simulink model "diffDrive"  (R2023a)
settings: Solver=VariableStepAuto  StartTime=0.0  StopTime=1  RelTol=1e-3
values from neighbouring files (symbols this model uses):
  ax = 0.1    [playground2.m]    (also in process_sim.m = [0, 0, 0.5, 0.5, 0.5, 0, 0, 0, -0.5, -0.5, -0.5])
  ax0 = 0    [process_sim.m]
  ay = 0.5    [playground2.m]    (also in process_sim.m = [0.25, 0.25, 0.25, 0.25, 0, 0, 0, 0, -0.75, -0.75, -0.75])
  ay0 = 0    [process_sim.m]
  fullX0 = [x0; y0; atan2(vy0, vx0); sqrt(vx0^2 + vy0^2); 0]    [playground2.m]    (also in process_sim.m = [x0; y0; atan2(vy0, vx0); sqrt(vx0^2 + vy0^2); 0] + delta)
  input_order = 2    [process_sim.m]
  jx = [0, 0, 1, 1, 1, -1, -1, -1, 0, 0, 0, -1, -1, -1, 1, 1, 1]    [process_sim.m]
  jy = [1, 1, 1, -1, -1, 0, 0, 0, -1, -1, -1, 1, 1, 1, 0, 0, 0]    [process_sim.m]
  T = 3    [playground.m]    (also in playground2.m = 0.1; predictiveControl.m = 0.1; process_sim.m = 0.1)
  vx0 = 0.5    [playground2.m]    (also in process_sim.m)
  vy0 = 0    [playground2.m]    (also in process_sim.m)
  x0 = x_lin + [0.01; -0.01; 0.02; 0.01; 0.001]    [playground.m]    (also in playground2.m = 0; process_sim.m = 0)
  y0 = 0    [playground2.m]    (also in process_sim.m)
settings Model: Creator=wcompton  LastModifiedBy=wcompton

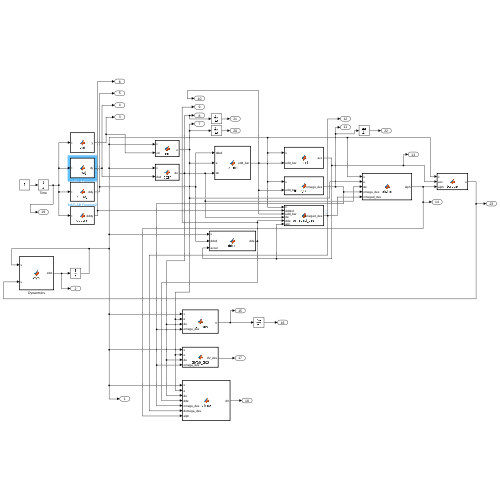
[thumbnail: Simulink's stored preview of the top-level diagram]
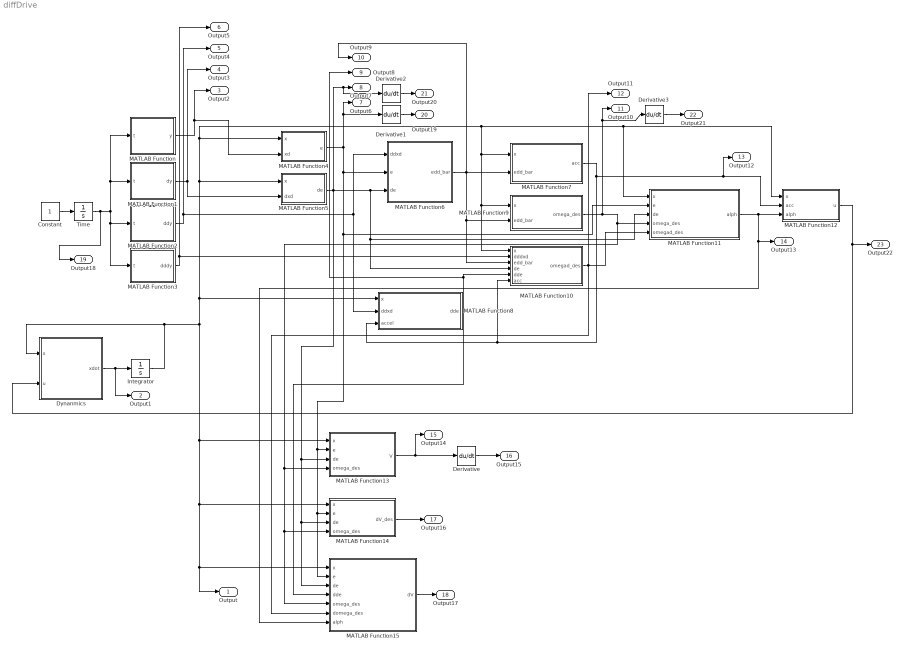
== system diffDrive ==
  Constant : Constant
  Derivative{,1..3} (4 alike) : Derivative
  Dynanmics : MATLAB Function  TreatAsAtomicUnit=on
  Integrator : Integrator  InitialCondition=fullX0
  MATLAB Function : MATLAB Function  TreatAsAtomicUnit=on
  MATLAB Function1 : MATLAB Function  TreatAsAtomicUnit=on
  MATLAB Function10 : MATLAB Function  TreatAsAtomicUnit=on
  MATLAB Function11 : MATLAB Function  TreatAsAtomicUnit=on
  MATLAB Function12 : MATLAB Function  TreatAsAtomicUnit=on
  MATLAB Function13 : MATLAB Function  TreatAsAtomicUnit=on
  MATLAB Function14 : MATLAB Function  TreatAsAtomicUnit=on
  MATLAB Function15 : MATLAB Function  TreatAsAtomicUnit=on
  MATLAB Function2 : MATLAB Function  TreatAsAtomicUnit=on
  MATLAB Function3 : MATLAB Function  TreatAsAtomicUnit=on
  MATLAB Function4 : MATLAB Function  TreatAsAtomicUnit=on
  MATLAB Function5 : MATLAB Function  TreatAsAtomicUnit=on
  MATLAB Function6 : MATLAB Function  TreatAsAtomicUnit=on
  MATLAB Function7 : MATLAB Function  TreatAsAtomicUnit=on
  MATLAB Function8 : MATLAB Function  TreatAsAtomicUnit=on
  MATLAB Function9 : MATLAB Function  TreatAsAtomicUnit=on
  Time : Integrator
  Output : Outport
  Output1 : Outport  Port=2
  Output2 : Outport  Port=3
  Output3 : Outport  Port=4
  Output4 : Outport  Port=5
  Output5 : Outport  Port=6
  Output6 : Outport  Port=7
  Output7 : Outport  Port=8
  Output8 : Outport  Port=9
  Output9 : Outport  Port=10
  Output10 : Outport  Port=11
  Output11 : Outport  Port=12
  Output12 : Outport  Port=13
  Output13 : Outport  Port=14
  Output14 : Outport  Port=15
  Output15 : Outport  Port=16
  Output16 : Outport  Port=17
  Output17 : Outport  Port=18
  Output18 : Outport  Port=19
  Output19 : Outport  Port=20
  Output20 : Outport  Port=21
  Output21 : Outport  Port=22
  Output22 : Outport  Port=23
  wires:
  Dynanmics/1(xdot) -> Integrator/1, Output1/1
  Integrator/1 -> MATLAB Function14/1(x), Output/1, MATLAB Function15/1(x), MATLAB Function13/1(x), MATLAB Function4/1(x), MATLAB Function9/1(x), MATLAB Function10/1(x), MATLAB Function7/1(x), MATLAB Function11/1(x), MATLAB Function12/1(x), MATLAB Function5/1(x), MATLAB Function8/1(x), Dynanmics/1(x)
  Constant/1 -> Time/1
  Time/1 -> Output18/1, MATLAB Function3/1(t), MATLAB Function2/1(t), MATLAB Function/1(t), MATLAB Function1/1(t)
  MATLAB Function/1(y) -> MATLAB Function4/2(xd), Output2/1
  MATLAB Function1/1(dy) -> Output3/1, MATLAB Function5/2(dxd)
  MATLAB Function4/1(e) -> MATLAB Function13/2(e), MATLAB Function15/2(e), MATLAB Function14/2(e), MATLAB Function11/2(e), MATLAB Function6/2(e), Derivative1/1, Output6/1
  MATLAB Function5/1(de) -> MATLAB Function6/3(de), MATLAB Function10/4(de), MATLAB Function11/3(de), Derivative2/1, Output7/1, MATLAB Function14/3(de), MATLAB Function15/3(de), MATLAB Function13/3(de)
  MATLAB Function2/1(ddy) -> Output4/1, MATLAB Function6/1(ddxd), MATLAB Function8/2(ddxd)
  MATLAB Function6/1(edd_bar) -> Output9/1, MATLAB Function9/2(edd_bar), MATLAB Function10/3(edd_bar), MATLAB Function7/2(edd_bar)
  MATLAB Function7/1(acc) -> MATLAB Function8/3(accel), MATLAB Function10/6(acc), Output12/1, MATLAB Function12/2(acc)
  MATLAB Function8/1(dde) -> MATLAB Function15/4(dde), MATLAB Function10/5(dde), Output8/1
  MATLAB Function9/1(omega_des) -> MATLAB Function11/4(omega_des), MATLAB Function13/4(omega_des), MATLAB Function14/4(omega_des), MATLAB Function15/5(omega_des), Output10/1, Derivative3/1
  MATLAB Function10/1(omegad_des) -> MATLAB Function15/6(domega_des), MATLAB Function11/5(omegad_des), Output11/1
  MATLAB Function11/1(alph) -> MATLAB Function15/7(alph), Output13/1, MATLAB Function12/3(alph)
  MATLAB Function12/1(u) -> Output22/1, Dynanmics/2(u)
  MATLAB Function13/1(V) -> Output14/1, Derivative/1
  MATLAB Function3/1(dddy) -> MATLAB Function10/2(dddxd), Output5/1
  MATLAB Function15/1(dV) -> Output17/1
  MATLAB Function14/1(dV_des) -> Output16/1
  Derivative/1 -> Output15/1
  Derivative1/1 -> Output19/1
  Derivative2/1 -> Output20/1
  Derivative3/1 -> Output21/1

== matlab function diffDrive/MATLAB Function6 ==
  data: ddxd input; edd_bar output; e input; de input; params parameter
function edd_bar = des_dde(ddxd, e, de, params)

edd_bar = ddxd - params.Kp * e - params.Kd * de;

== matlab function diffDrive/MATLAB Function7 ==
  data: x input; acc output; edd_bar input
function acc = accel(x, edd_bar)

acc = [cos(x(3)), sin(x(3))] * edd_bar;

== matlab function diffDrive/MATLAB Function8 ==
  data: x input; dde output; ddxd input; accel input
function dde = dderr(x, ddxd, accel)

dde = - ddxd + [cos(x(3)), -x(4) * sin(x(3)); sin(x(3)), x(4) * cos(x(3))] * [accel; x(5)];

== matlab function diffDrive/MATLAB Function9 ==
  data: x input; omega_des output; edd_bar input
function omega_des = omega_des(x, edd_bar)

omega_des = [-1 / x(4) * sin(x(3)), 1 / x(4) * cos(x(3))] * edd_bar;

== matlab function diffDrive/MATLAB Function10 ==
  data: x input; dddxd input; omegad_des output; edd_bar input; de input; dde input; acc input; params parameter
function omegad_des = omegad_des(x, dddxd, edd_bar, de, dde, acc, params)

omegad_des = [acc / x(4)^2 * sin(x(3)) - x(5) / x(4) * cos(x(3)), -acc / x(4)^2 * cos(x(3)) - x(5) / x(4) * sin(x(3))] * edd_bar + [-1 / x(4) * sin(x(3)), 1 / x(4) * cos(x(3))] * (dddxd - params.Kp * de - params.Kd * dde);

== matlab function diffDrive/MATLAB Function11 ==
  data: x input; e input; de input; alph output; omega_des input; omegad_des input; params parameter
function alph = alpha(x, e, de, omega_des, omegad_des, params)

alph = -params.sigma / 2 * (x(5) - omega_des) + omegad_des - 2 * [e', de'] * params.P * [0; 0; -x(4) * sin(x(3)); x(4) * cos(x(3))];

== matlab function diffDrive/MATLAB Function12 ==
  data: x input; u output; acc input; alph input; params parameter
function u = torque(x, acc, alph, params)

u = accelToTorque(x, [acc; alph], params);

== matlab function diffDrive/MATLAB Function13 ==
  data: x input; V output; e input; de input; omega_des input; params parameter
function V = laypunov(x, e, de, omega_des, params)

Ve = [e; de]' * params.P * [e; de];
V = Ve + 0.5 * (omega_des - x(5)).^2;

== matlab function diffDrive/MATLAB Function14 ==
  data: x input; dV_des output; e input; de input; omega_des input; params parameter
function dV_des = dlyap_des(x, e, de, omega_des, params)

dVe = -[e; de]' * [e; de];
dV_des = dVe - params.sigma / 2 * (omega_des - x(5)).^2;

== matlab function diffDrive/MATLAB Function ==
  data: t input; y output; x0 parameter; vx0 parameter; ax0 parameter; y0 parameter; vy0 parameter; ay0 parameter; T parameter; ax parameter; ay parameter; jx parameter; jy parameter; input_order parameter
function y = traj(t, x0, vx0, ax0, y0, vy0, ay0, T, ax, ay, jx, jy, input_order)
if input_order == 2
    ind = 1;
    while t > T
        x0 = x0 + vx0 * T + 0.5 * ax(ind) * T^2;
        vx0 = vx0 + ax(ind) * T;
        y0 = y0 + vy0 * T + 0.5 * ay(ind) * T^2;
        vy0 = vy0 + ay(ind) * T;
        t = t - T;
        ind = ind + 1;
    end
    y = [x0 + vx0 * t + 0.5 * ax(ind) * t^2;y0 + vy0 * t + 0.5 * ay(ind) * t^2];
elseif input_order == 3
    ind = 1;
    while t > T
        x0 = x0 + vx0 * T + 0.5 * ax0 * T^2 + 1/6 * jx(ind) * T^3;
        vx0 = vx0 + ax0 * T + 0.5 * jx(ind) * T^2;
        ax0 = ax0 + jx(ind) * T;
        y0 = y0 + vy0 * T + 0.5 * ay0 * T^2 + 1/6 * jy(ind) * T^3;
        vy0 = vy0 + ay0 * T + 0.5 * jy(ind) * T^2;
        ay0 = ay0 + jy(ind) * T;
        t = t - T;
        ind = ind + 1;
    end
    y = [x0 + vx0 * t + 0.5 * ax0 * t^2 + jx(ind) / 6 * t^3; y0 + vy0 * t + 0.5 * ay0 * t^2 + jy(ind) / 6 * t^3];
else
    y = [0; 0];
end

== matlab function diffDrive/MATLAB Function15 ==
  data: x input; dV output; e input; de input; dde input; omega_des input; domega_des input; alph input; params parameter
function dV = dlyap(x, e, de, dde, omega_des, domega_des, alph, params)

dV = 2 * [de; dde]' * params.P * [e; de] + (omega_des - x(5)) * (domega_des - alph);

== matlab function diffDrive/Dynanmics ==
  data: x input; u input; xdot output; params parameter
function xdot = dyn(x, u, params)

th = x(3);
v = x(4);
w = x(5);
R = params.R;
L = params.L;
alpha = params.m + 2 * params.Iw / R.^2;
beta = params.I + 2 * L^.2 / R.^2 * params.Iw;
mcd = params.mc * params.d;

tr = u(1);
tl = u(2);

xdot = [
    v * cos(th);
    v * sin(th);
    w;
    (mcd * w.^2 + (tr + tl) / R) / alpha;
    (-mcd * w * v + (tr - tl) * L / R) / beta
];

== matlab function diffDrive/MATLAB Function1 ==
  data: t input; dy output; vx0 parameter; ax0 parameter; vy0 parameter; ay0 parameter; T parameter; ax parameter; ay parameter; jx parameter; jy parameter; input_order parameter
function dy = dtraj(t, vx0, ax0, vy0, ay0, T, ax, ay, jx, jy, input_order)
if input_order == 2
    ind = 1;
    while t > T
        vx0 = vx0 + ax(ind) * T;
        vy0 = vy0 + ay(ind) * T;
        t = t - T;
        ind = ind + 1;
    end
    dy = [vx0 + ax(ind) * t; vy0 + ay(ind) * t];
elseif input_order == 3
    ind = 1;
    while t > T
        vx0 = vx0 + ax0 * T + 0.5 * jx(ind) * T^2;
        ax0 = ax0 + jx(ind) * T;
        vy0 = vy0 + ay0 * T + 0.5 * jy(ind) * T^2;
        ay0 = ay0 + jy(ind) * T;
        t = t - T;
        ind = ind + 1;
    end
    dy = [vx0 + ax0 * t + jx(ind) / 2 * t^2; vy0 + ay0 * t + jy(ind) / 2 * t^2];
else 
    dy = [0; 0];
end

== matlab function diffDrive/MATLAB Function2 ==
  data: t input; ddy output; ax0 parameter; ay0 parameter; T parameter; ax parameter; ay parameter; jx parameter; jy parameter; input_order parameter
function ddy = ddtraj(t, ax0, ay0, T, ax, ay, jx, jy, input_order)
if input_order == 2
    ind = 1;
    while t > T
        t = t - T;
        ind = ind + 1;
    end
    ddy = [ax(ind); ay(ind)];
elseif input_order == 3
    ind = 1;
    while t > T
        ax0 = ax0 + jx(ind) * T;
        ay0 = ay0 + jy(ind) * T;
        t = t - T;
        ind = ind + 1;
    end
    ddy = [ax0 + jx(ind) * t; ay0 + jy(ind) * t];
else
    ddy = [0; 0];
end

== matlab function diffDrive/MATLAB Function3 ==
  data: t input; dddy output; T parameter; jx parameter; jy parameter; input_order parameter
function dddy = dddtraj(t, T, jx, jy, input_order)
if input_order == 2
    dddy = [0; 0];
elseif input_order == 3
    ind = 1;
    while t > T
        t = t - T;
        ind = ind + 1;
    end
    dddy = [jx(ind); jy(ind)];
else
    dddy = [0; 0];
end

== matlab function diffDrive/MATLAB Function4 ==
  data: x input; e output; xd input
function e = err(x, xd)
e = x(1:2) - xd;

== matlab function diffDrive/MATLAB Function5 ==
  data: x input; de output; dxd input
function de = derr(x, dxd)
de = x(4) * [cos(x(3)); sin(x(3))] - dxd;
